simulink model "Pacemaker"  (R2020a)
settings: Solver=FixedStepAuto  StartTime=0.0  StopTime=inf  FixedStep=1e-3  RelTol=1e-3  EnableMultiTasking=on
undefined symbols (not defined in the file): A0, A1, D0, D1, D10, D11, D12, D13, D2, D3, D4, D5, D6, D7, D8, D9, magnitude, PTA0, PTA1, PTA2, PTB2, PTB23, PTB3, PTB9, PTC16, PTC17, PTC2, PTC3, PTC4, PTD0, PTD1, PTD2, PTD3
libraries: frdmk64flib x22, etargetslib x22
settings Model: ExtModeTrigDuration=5  Creator=ffara  LastModifiedBy=Usman Minhas
settings OptimizationCC: EnhancedBackFolding=on  PassReuseOutputArgsAs=Individual arguments  ZeroExternalMemoryAtStartup=off  ZeroInternalMemoryAtStartup=off  MaxStackSize=64  OptimizeBlockOrder=speed  DifferentSizesBufferReuse=on  OptimizationCustomize=off  EfficientTunableParamExpr=on
settings DebuggingCC: ParameterTunabilityLossMsg=error
settings HardwareCC: ProdBitPerPointer=32  ProdBitPerSizeT=32  ProdBitPerPtrDiffT=32  ProdLargestAtomicInteger=Long  ProdLargestAtomicFloat=Double  ProdWordSize=32  ProdHWDeviceType=ARM Compatible->ARM Cortex
settings SFSimCC: MATLABDynamicMemAlloc=off
settings RTWCC: SystemTargetFile=ert.tlc  HardwareBoard=NXP FRDM-K64F  TemplateMakefile=ert_default_tmf  Toolchain=GNU Tools for ARM Embedded Processors
settings CodeAppCC: ForceParamTrailComments=on  IgnoreCustomStorageClasses=off  OperatorAnnotations=on  SimulinkDataObjDesc=on  SFDataObjDesc=on  InsertBlockDesc=on

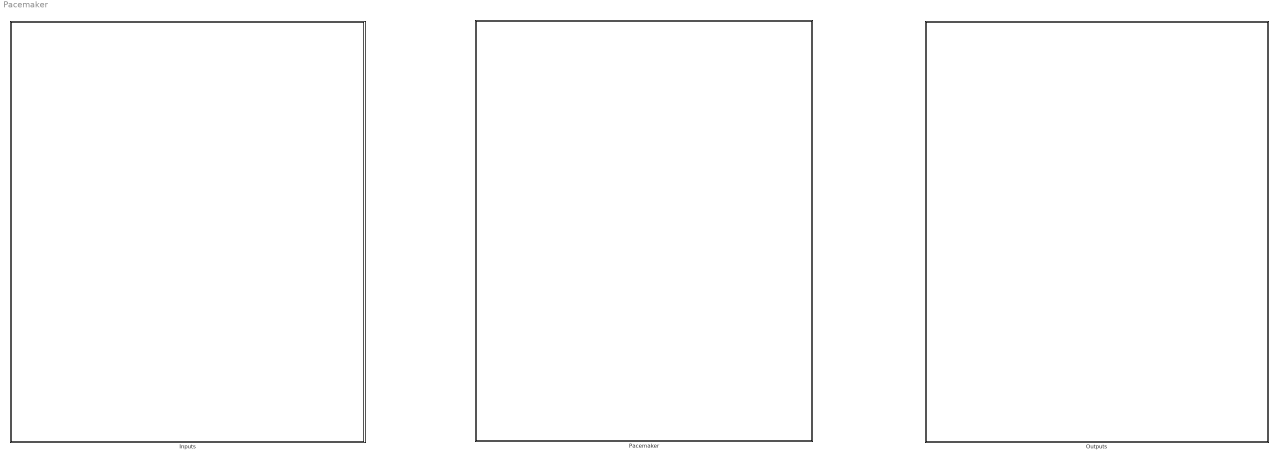
== system Pacemaker ==
  Inputs : Subsystem
  Outputs : Subsystem
  Pacemaker : Subsystem

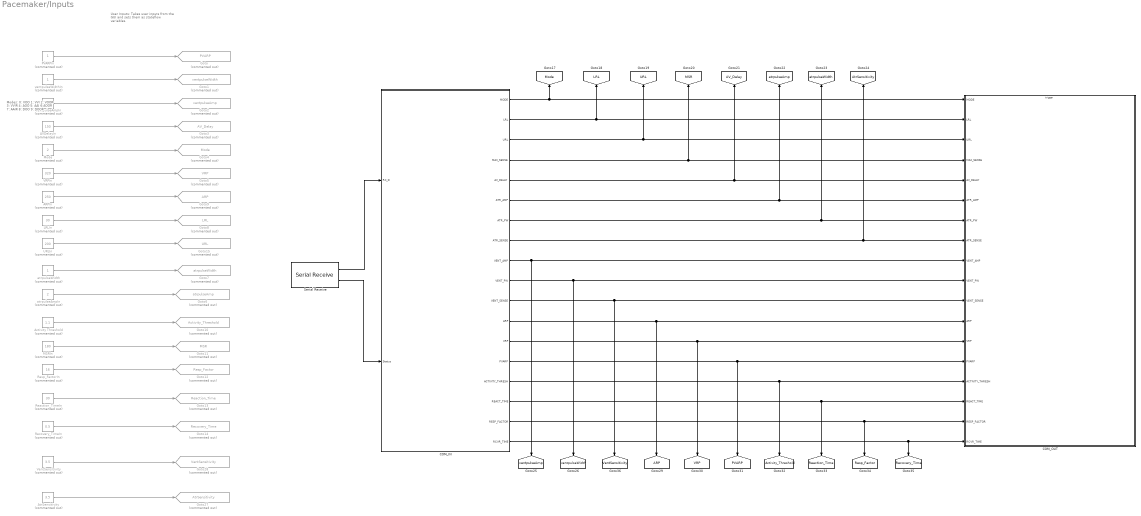
== system Pacemaker/Inputs ==
  note: User Inputs:
      | Takes user inputs from the GUI and sets them as stateflow variables.
  note: Modes:
      | 0: VOO
      | 1: VVI
      | 2: VOOR
      | 3: VVIR
      | 4: AOO
      | 5: AAI
      | 6:AOOR
      | 7: AAIR
      | 8: DOO
      | 9: DOOR
  ARPIn : Constant  Commented=on  Value=250
  AVDelayIn : Constant  Commented=on  Value=150
  Activity Threshold : Constant  Commented=on  Value=1.1
  AtrSensitivity : Constant  Commented=on  Value=3.5
  COM_IN : Stateflow chart  TreatAsAtomicUnit=on
  COM_OUT : Subsystem
  Goto : Goto  Commented=on  GotoTag=PVARP  TagVisibility=global
  Goto1 : Goto  Commented=on  GotoTag=ventpulseWidth  TagVisibility=global
  Goto10 : Goto  Commented=on  GotoTag=Activity_Threshold  TagVisibility=global
  Goto11 : Goto  Commented=on  GotoTag=MSR  TagVisibility=global
  Goto12 : Goto  Commented=on  GotoTag=Resp_Factor  TagVisibility=global
  Goto13 : Goto  Commented=on  GotoTag=Reaction_Time  TagVisibility=global
  Goto14 : Goto  Commented=on  GotoTag=Recovery_Time  TagVisibility=global
  Goto15 : Goto  Commented=on  GotoTag=URL  TagVisibility=global
  Goto2 : Goto  Commented=on  GotoTag=ventpulseAmp  TagVisibility=global
  Goto27 : Goto  Commented=on  GotoTag=AtrSensitivity  TagVisibility=global
  Goto28 : Goto  Commented=on  GotoTag=VentSensitivity  TagVisibility=global
  Goto3 : Goto  Commented=on  GotoTag=AV_Delay  TagVisibility=global
  Goto4 : Goto  Commented=on  GotoTag=Mode  TagVisibility=global
  Goto5 : Goto  Commented=on  GotoTag=VRP  TagVisibility=global
  Goto6 : Goto  Commented=on  GotoTag=atrpulseAmp  TagVisibility=global
  Goto7 : Goto  Commented=on  GotoTag=atrpulseWidth  TagVisibility=global
  Goto8 : Goto  Commented=on  GotoTag=LRL  TagVisibility=global
  Goto9 : Goto  Commented=on  GotoTag=ARP  TagVisibility=global
  LRLIn : Constant  Commented=on  Value=30
  MSRIn : Constant  Commented=on  Value=180
  Mode : Constant  Commented=on  Value=2
  PVARPIn : Constant  Commented=on
  Reaction_TimeIn : Constant  Commented=on  Value=30
  Recovery_TimeIn : Constant  Commented=on  Value=0.5
  Resp_FactorIn : Constant  Commented=on  Value=16
  Serial Receive : frdmk64flib/Serial Receive  SCIModule=0  Baudrate=uint32(9600)  Parity=None  StopBits=1  HardwareFlowControl=None  ByteOrder=LittleEndian  DataType=uint8  DataLength=68  BlockingMode=off  OutputStatus=on  SampleTime=-1
  URLIn : Constant  Commented=on  Value=200
  VRPIn : Constant  Commented=on  Value=320
  VentSensitivity : Constant  Commented=on  Value=3.5
  atrpulseAmpIn : Constant  Commented=on  Value=2
  atrpulseWidth : Constant  Commented=on
  ventpulseAmpIn : Constant  Commented=on  Value=5
  ventpulseWidthIn : Constant  Commented=on
  tag scope: ARP=global, AV_Delay=global, Activity_Threshold=global, AtrSensitivity=global, LRL=global, MSR=global, Mode=global, PVARP=global, Reaction_Time=global, Recovery_Time=global, Resp_Factor=global, URL=global, VRP=global, VentSensitivity=global, atrpulseAmp=global, atrpulseWidth=global, ventpulseAmp=global, ventpulseWidth=global
  wires:
  Resp_FactorIn/1 -> Goto12/1
  PVARPIn/1 -> Goto/1
  VRPIn/1 -> Goto5/1
  ventpulseWidthIn/1 -> Goto1/1
  LRLIn/1 -> Goto8/1
  VentSensitivity/1 -> Goto28/1
  Mode/1 -> Goto4/1
  AtrSensitivity/1 -> Goto27/1
  URLIn/1 -> Goto15/1
  atrpulseWidth/1 -> Goto7/1
  AVDelayIn/1 -> Goto3/1
  ARPIn/1 -> Goto9/1
  atrpulseAmpIn/1 -> Goto6/1
  ventpulseAmpIn/1 -> Goto2/1
  Activity Threshold/1 -> Goto10/1
  Reaction_TimeIn/1 -> Goto13/1
  Recovery_TimeIn/1 -> Goto14/1
  MSRIn/1 -> Goto11/1
  Serial Receive/2 -> COM_IN/2(Status)
  COM_IN/1(MODE) -> [Mode], COM_OUT/1(MODE)
  Serial Receive/1 -> COM_IN/1(RX_D)
  COM_IN/2(LRL) -> [LRL], COM_OUT/2(LRL)
  COM_IN/3(URL) -> [URL], COM_OUT/3(URL)
  COM_IN/4(MAX_SENSE) -> [MSR], COM_OUT/4(MAX_SENSE)
  COM_IN/5(AV_DELAY) -> [AV_Delay], COM_OUT/5(AV_DELAY)
  COM_IN/6(ATR_AMP) -> [atrpulseAmp], COM_OUT/6(ATR_AMP)
  COM_IN/7(ATR_PW) -> [atrpulseWidth], COM_OUT/7(ATR_PW)
  COM_IN/8(ATR_SENSE) -> [AtrSensitivity], COM_OUT/8(ATR_SENSE)
  COM_IN/9(VENT_AMP) -> [ventpulseAmp], COM_OUT/9(VENT_AMP)
  COM_IN/10(VENT_PW) -> COM_OUT/10(VENT_PW), [ventpulseWidth]
  COM_IN/11(VENT_SENSE) -> [VentSensitivity], COM_OUT/11(VENT_SENSE)
  COM_IN/12(ARP) -> COM_OUT/12(ARP), [ARP]
  COM_IN/13(VRP) -> [VRP], COM_OUT/13(VRP)
  COM_IN/14(PVARP) -> [PVARP], COM_OUT/14(PVARP)
  COM_IN/15(ACTIVITY_THRESH) -> [Activity_Threshold], COM_OUT/15(ACTIVITY_THRESH)
  COM_IN/16(REACT_TIME) -> [Reaction_Time], COM_OUT/16(REACT_TIME)
  COM_IN/17(RESP_FACTOR) -> [Resp_Factor], COM_OUT/17(RESP_FACTOR)
  COM_IN/18(RCVR_TIME) -> [Recovery_Time], COM_OUT/18(RCVR_TIME)

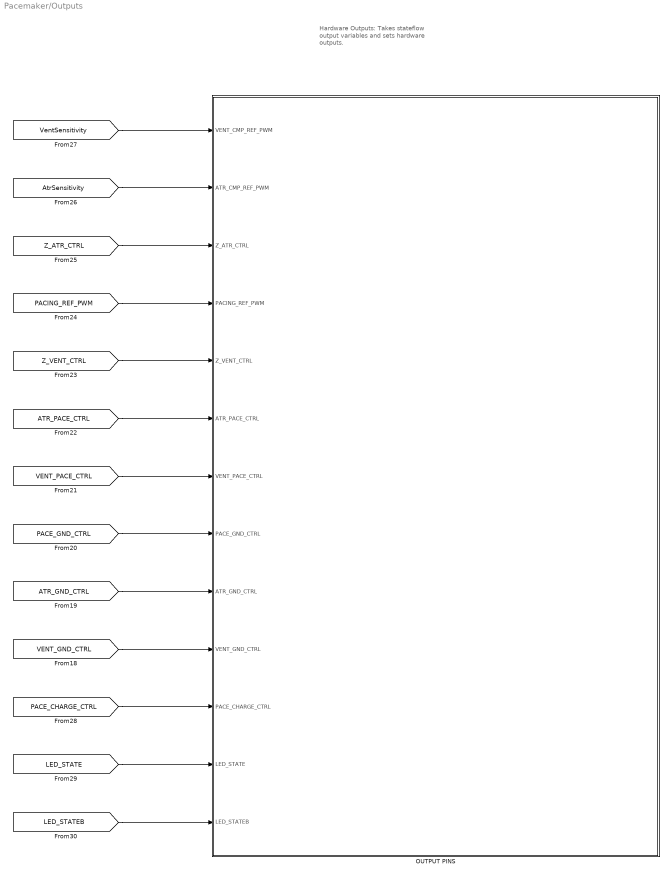
== system Pacemaker/Outputs ==
  note: Hardware Outputs:
      | Takes stateflow output variables and sets hardware outputs.
  OUTPUT PINS : Subsystem
  wires:
  [VentSensitivity] -> OUTPUT PINS/1(VENT_CMP_REF_PWM)
  [PACE_CHARGE_CTRL] -> OUTPUT PINS/11(PACE_CHARGE_CTRL)
  [ATR_PACE_CTRL] -> OUTPUT PINS/6(ATR_PACE_CTRL)
  [LED_STATEB] -> OUTPUT PINS/13(LED_STATEB)
  [LED_STATE] -> OUTPUT PINS/12(LED_STATE)
  [PACING_REF_PWM] -> OUTPUT PINS/4(PACING_REF_PWM)
  [AtrSensitivity] -> OUTPUT PINS/2(ATR_CMP_REF_PWM)
  [Z_ATR_CTRL] -> OUTPUT PINS/3(Z_ATR_CTRL)
  [PACE_GND_CTRL] -> OUTPUT PINS/8(PACE_GND_CTRL)
  [VENT_PACE_CTRL] -> OUTPUT PINS/7(VENT_PACE_CTRL)
  [ATR_GND_CTRL] -> OUTPUT PINS/9(ATR_GND_CTRL)
  [Z_VENT_CTRL] -> OUTPUT PINS/5(Z_VENT_CTRL)
  [VENT_GND_CTRL] -> OUTPUT PINS/10(VENT_GND_CTRL)

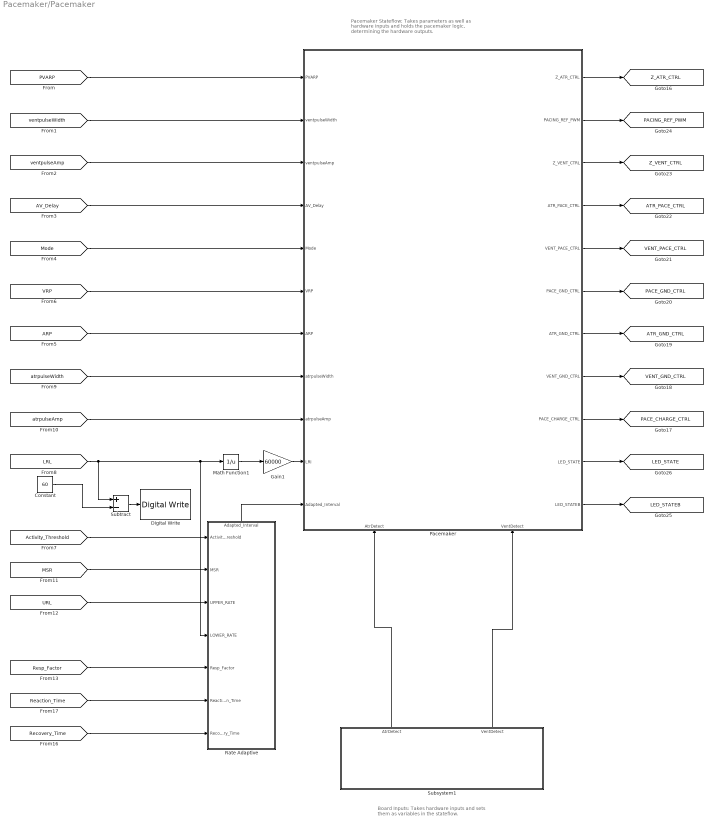
== system Pacemaker/Pacemaker ==
  note: Board Inputs:
      | Takes hardware inputs and sets them as variables in the stateflow.
  note: Pacemaker Stateflow:
      | Takes parameters as well as hardware inputs
      | and holds the pacemaker logic, determining the hardware outputs.
  Constant : Constant  Value=60
  Digital Write : frdmk64flib/Digital Write  Whichpin=GREEN_LED
  Gain1 : Gain  Gain=60000  RndMeth=Ceiling
  Math Function1 : Math  Operator=reciprocal  OutputSignalType=real  OutDataTypeStr=double  RndMeth=Ceiling  SaturateOnIntegerOverflow=on
  Pacemaker : Stateflow chart  TreatAsAtomicUnit=on
      settings: PortSchema="{\"entries\":[{\"content\":{\"sides\":[{\"content\":{\"connectorIds\":[\"In1\",\"In10\",\"In3\",\"In4\",\"In6\",\"In7\",\"In8\",\"In9\",\"In13\",\"In12\",\"In11\"]},\"type\":\"ConnectorPlacement.EquallySpacedRectSide\",\"uuid\":\"aed163b7-0e0a-4c56-a109-22d9582f06bc\"},{\"content\":{\"connectorIds\":[\"Out1\",\"Out3\",\"Out2\",\"Out4\",\"Out5\",\"Out6\",\"Out7\",\"Out8\",\"Out9\",\"Out10\",\"Out11\"],\"side\":\"RIGHT\"},\"type\":\"ConnectorPlacement.EquallySpacedRectSide\",\"uuid\":\"7c994607-95c8-4912-b49a-f01b42451ae0\"},{\"content\":{\"connectorIds\":[],\"side\":\"TOP\"},\"type\":\"ConnectorPlacement.EquallySpacedRectSide\",\"uuid\":\"6d27b0f7-5c71-41f2-b80a-818ae3f7f3ce\"},{\"content\":{\"connectorIds\":[\"In2\",\"In5\"],\"side\":\"BOTTOM\"},\"type\":\"ConnectorPlacement.EquallySpacedRectSide\",\"uuid\":\"17f29399-4528-40af-8d63-94f1f3c418c0\"}]},\"type\":\"ConnectorPlacement.EquallySpacedConnector\",\"uuid\":\"6ca6b560-67cc-4d2d-81f4-cc3fe3468b1a\"}],\"packageUris\":[\"http://schema.mathworks.com/mf0/Connector/19700101\"],\"version\":\"1.0\"}"
  Rate Adaptive : Subsystem
      settings: PortSchema="{\"entries\":[{\"content\":{\"sides\":[{\"content\":{\"connectorIds\":[\"In1\",\"In2\",\"In3\",\"In4\",\"In5\",\"In6\",\"In7\"]},\"type\":\"ConnectorPlacement.EquallySpacedRectSide\",\"uuid\":\"c17ee6c3-7042-4555-a185-2b3f1c7c5c48\"},{\"content\":{\"connectorIds\":[],\"side\":\"RIGHT\"},\"type\":\"ConnectorPlacement.EquallySpacedRectSide\",\"uuid\":\"ce834616-f3de-4ad9-afed-1295335ec238\"},{\"content\":{\"connectorIds\":[\"Out1\"],\"side\":\"TOP\"},\"type\":\"ConnectorPlacement.EquallySpacedRectSide\",\"uuid\":\"ee6be2e3-da9a-4870-9d5e-446ab0e3551d\"}]},\"type\":\"ConnectorPlacement.EquallySpacedConnector\",\"uuid\":\"5402bfdc-705b-4da9-91cb-a8abac72fcc2\"}],\"packageUris\":[\"http://schema.mathworks.com/mf0/Connector/19700101\"],\"version\":\"1.0\"}"
  Subsystem1 : Subsystem
      settings: PortSchema="{\"entries\":[{\"content\":{\"sides\":[{\"content\":{\"connectorIds\":[]},\"type\":\"ConnectorPlacement.EquallySpacedRectSide\",\"uuid\":\"29534348-9b3e-49a9-890e-1782155d7d1f\"},{\"content\":{\"connectorIds\":[],\"side\":\"RIGHT\"},\"type\":\"ConnectorPlacement.EquallySpacedRectSide\",\"uuid\":\"db3d28f5-8266-45b6-9ee4-e43788b67d28\"},{\"content\":{\"connectorIds\":[\"Out1\",\"Out2\"],\"side\":\"TOP\"},\"type\":\"ConnectorPlacement.EquallySpacedRectSide\",\"uuid\":\"67bf6cf6-8ed6-4181-b5d9-914949d467ab\"}]},\"type\":\"ConnectorPlacement.EquallySpacedConnector\",\"uuid\":\"34dda7e8-1d86-47a2-be1a-f2253f8f1257\"}],\"packageUris\":[\"http://schema.mathworks.com/mf0/Connector/R2020b\"],\"version\":\"1.0\"}"
  Subtract : Sum  Inputs=+-
  tag scope: ATR_GND_CTRL=global, ATR_PACE_CTRL=global, LED_STATE=global, LED_STATEB=global, PACE_CHARGE_CTRL=global, PACE_GND_CTRL=global, PACING_REF_PWM=global, VENT_GND_CTRL=global, VENT_PACE_CTRL=global, Z_ATR_CTRL=global, Z_VENT_CTRL=global
  wires:
  Pacemaker/7(ATR_GND_CTRL) -> [ATR_GND_CTRL]
  Subsystem1/1(AtrDetect) -> Pacemaker/2(AtrDetect)
  Pacemaker/4(ATR_PACE_CTRL) -> [ATR_PACE_CTRL]
  Pacemaker/10(LED_STATE) -> [LED_STATE]
  [AV_Delay] -> Pacemaker/4(AV_Delay)
  Pacemaker/2(Z_VENT_CTRL) -> [Z_VENT_CTRL]
  [Mode] -> Pacemaker/6(Mode)
  [ARP] -> Pacemaker/8(ARP)
  Pacemaker/1(Z_ATR_CTRL) -> [Z_ATR_CTRL]
  Math Function1/1 -> Gain1/1
  [atrpulseWidth] -> Pacemaker/9(atrpulseWidth)
  [PVARP] -> Pacemaker/1(PVARP)
  Pacemaker/5(VENT_PACE_CTRL) -> [VENT_PACE_CTRL]
  Pacemaker/6(PACE_GND_CTRL) -> [PACE_GND_CTRL]
  Pacemaker/11(LED_STATEB) -> [LED_STATEB]
  [Resp_Factor] -> Rate Adaptive/5(Resp_Factor)
  Pacemaker/3(PACING_REF_PWM) -> [PACING_REF_PWM]
  [MSR] -> Rate Adaptive/2(MSR)
  [ventpulseWidth] -> Pacemaker/10(ventpulseWidth)
  Pacemaker/8(VENT_GND_CTRL) -> [VENT_GND_CTRL]
  Pacemaker/9(PACE_CHARGE_CTRL) -> [PACE_CHARGE_CTRL]
  [ventpulseAmp] -> Pacemaker/3(ventpulseAmp)
  [Recovery_Time] -> Rate Adaptive/7(Recovery_Time)
  Subsystem1/2(VentDetect) -> Pacemaker/5(VentDetect)
  [URL] -> Rate Adaptive/3(UPPER_RATE)
  [atrpulseAmp] -> Pacemaker/13(atrpulseAmp)
  Gain1/1 -> Pacemaker/12(LRI)
  [VRP] -> Pacemaker/7(VRP)
  [Activity_Threshold] -> Rate Adaptive/1(Activity_Threshold)
  [LRL] -> Subtract/1, Math Function1/1, Rate Adaptive/4(LOWER_RATE)
  Rate Adaptive/1(Adapted_Interval) -> Pacemaker/11(Adapted_Interval)
  [Reaction_Time] -> Rate Adaptive/6(Reaction_Time)
  Subtract/1 -> Digital Write/1
  Constant/1 -> Subtract/2

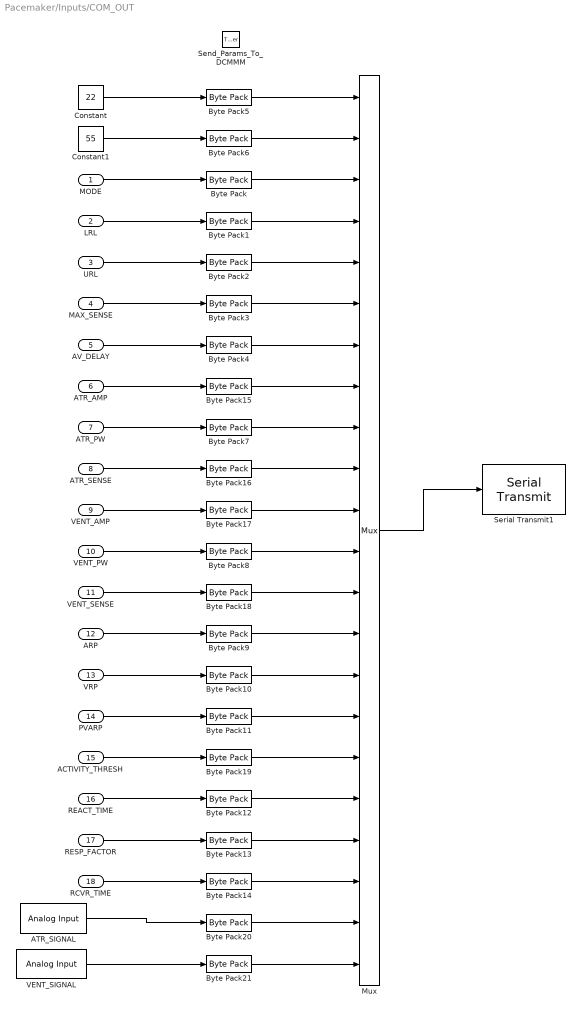
== system Pacemaker/Inputs/COM_OUT ==
  MODE : Inport
  LRL : Inport  Port=2
  URL : Inport  Port=3
  MAX_SENSE : Inport  Port=4
  AV_DELAY : Inport  Port=5
  ATR_AMP : Inport  Port=6
  ATR_PW : Inport  Port=7
  ATR_SENSE : Inport  Port=8
  VENT_AMP : Inport  Port=9
  VENT_PW : Inport  Port=10
  VENT_SENSE : Inport  Port=11
  ARP : Inport  Port=12
  VRP : Inport  Port=13
  PVARP : Inport  Port=14
  ACTIVITY_THRESH : Inport  Port=15
  REACT_TIME : Inport  Port=16
  RESP_FACTOR : Inport  Port=17
  RCVR_TIME : Inport  Port=18
  Send_Params_To_DCMMM : TriggerPort  TriggerType=function-call  IsSimulinkFunction=on  FunctionName=Send_Params_To_DCMMM  VariantControl=Variant
  ATR_SIGNAL : frdmk64flib/Analog Input  Whichpin=PTB2 (A0)  SampleTime=-1
  Byte Pack{,1..4,7..14} (13 alike) : etargetslib/Byte Pack  datatypes={'uint16'}  byteAlign=1
  Byte Pack{15..21} (7 alike) : etargetslib/Byte Pack  datatypes={'double'}  byteAlign=1
  Byte Pack5 : etargetslib/Byte Pack  datatypes={'uint8'}  byteAlign=1
  Byte Pack6 : etargetslib/Byte Pack  datatypes={'uint8'}  byteAlign=1
  Constant : Constant  Value=22  OutDataTypeStr=uint8
  Constant1 : Constant  Value=55  OutDataTypeStr=uint8
  Mux : Mux  Inputs=22
  Serial Transmit1 : frdmk64flib/Serial Transmit  SCIModule=0  Baudrate=uint32(9600)  Parity=None  StopBits=1  HardwareFlowControl=None  ByteOrder=LittleEndian  BlockingMode=on  OutputStatus=off
  VENT_SIGNAL : frdmk64flib/Analog Input  Whichpin=PTB3 (A1)  SampleTime=-1
  wires:
  Mux/1 -> Serial Transmit1/1
  MODE/1 -> Byte Pack/1
  Byte Pack/1 -> Mux/3
  Constant/1 -> Byte Pack5/1
  Byte Pack5/1 -> Mux/1
  Byte Pack6/1 -> Mux/2
  Constant1/1 -> Byte Pack6/1
  Byte Pack1/1 -> Mux/4
  Byte Pack2/1 -> Mux/5
  Byte Pack3/1 -> Mux/6
  Byte Pack4/1 -> Mux/7
  URL/1 -> Byte Pack2/1
  MAX_SENSE/1 -> Byte Pack3/1
  AV_DELAY/1 -> Byte Pack4/1
  RCVR_TIME/1 -> Byte Pack14/1
  RESP_FACTOR/1 -> Byte Pack13/1
  REACT_TIME/1 -> Byte Pack12/1
  Byte Pack12/1 -> Mux/18
  Byte Pack13/1 -> Mux/19
  Byte Pack14/1 -> Mux/20
  Byte Pack9/1 -> Mux/14
  Byte Pack10/1 -> Mux/15
  Byte Pack11/1 -> Mux/16
  PVARP/1 -> Byte Pack11/1
  VRP/1 -> Byte Pack10/1
  ARP/1 -> Byte Pack9/1
  Byte Pack7/1 -> Mux/9
  Byte Pack8/1 -> Mux/12
  VENT_PW/1 -> Byte Pack8/1
  ATR_PW/1 -> Byte Pack7/1
  LRL/1 -> Byte Pack1/1
  Byte Pack19/1 -> Mux/17
  Byte Pack17/1 -> Mux/11
  Byte Pack16/1 -> Mux/10
  Byte Pack15/1 -> Mux/8
  Byte Pack18/1 -> Mux/13
  ATR_AMP/1 -> Byte Pack15/1
  ATR_SENSE/1 -> Byte Pack16/1
  VENT_AMP/1 -> Byte Pack17/1
  VENT_SENSE/1 -> Byte Pack18/1
  ACTIVITY_THRESH/1 -> Byte Pack19/1
  ATR_SIGNAL/1 -> Byte Pack20/1
  VENT_SIGNAL/1 -> Byte Pack21/1
  Byte Pack20/1 -> Mux/21
  Byte Pack21/1 -> Mux/22

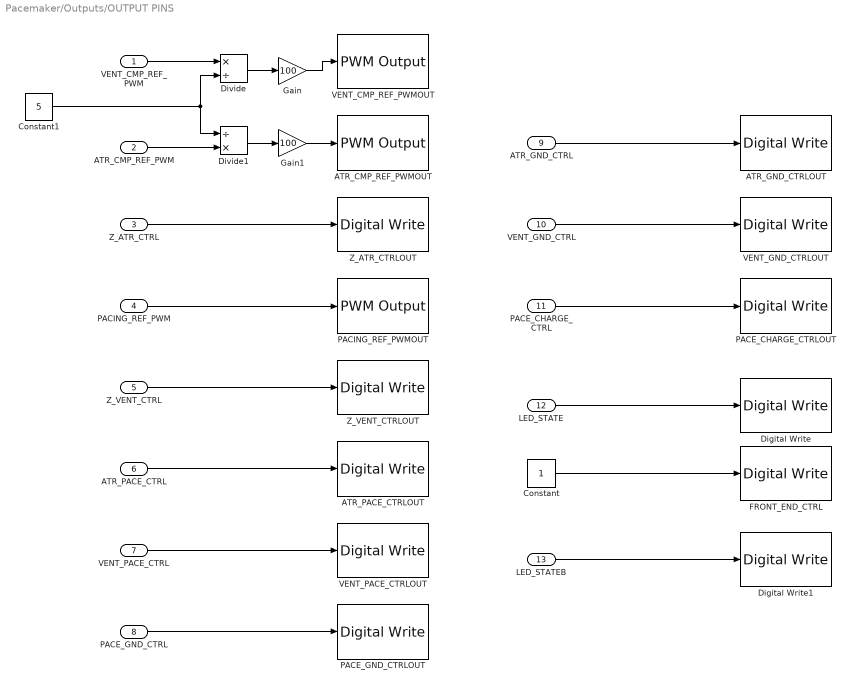
== system Pacemaker/Outputs/OUTPUT PINS ==
  VENT_CMP_REF_PWM : Inport  Unit=mV
  ATR_CMP_REF_PWM : Inport  Port=2  Unit=mV
  Z_ATR_CTRL : Inport  Port=3
  PACING_REF_PWM : Inport  Port=4
  Z_VENT_CTRL : Inport  Port=5
  ATR_PACE_CTRL : Inport  Port=6
  VENT_PACE_CTRL : Inport  Port=7
  PACE_GND_CTRL : Inport  Port=8
  ATR_GND_CTRL : Inport  Port=9
  VENT_GND_CTRL : Inport  Port=10
  PACE_CHARGE_CTRL : Inport  Port=11
  LED_STATE : Inport  Port=12
  LED_STATEB : Inport  Port=13
  ATR_CMP_REF_PWMOUT : frdmk64flib/PWM Output  Whichpin=PTC2 (D6)  InitialFrequency=2000  InitialDutyCycle=0
  ATR_GND_CTRLOUT : frdmk64flib/Digital Write  Whichpin=PTD2 (D11)
  ATR_PACE_CTRLOUT : frdmk64flib/Digital Write  Whichpin=PTA0 (D8)
  Constant : Constant
  Constant1 : Constant  Value=5
  Digital Write : frdmk64flib/Digital Write  Whichpin=RED_LED
  Digital Write1 : frdmk64flib/Digital Write  Whichpin=BLUE_LED
  Divide : Product  Inputs=*/
  Divide1 : Product  Inputs=/*
  FRONT_END_CTRL : frdmk64flib/Digital Write  Whichpin=PTD1 (D13)
  Gain : Gain  Gain=100
  Gain1 : Gain  Gain=100
  PACE_CHARGE_CTRLOUT : frdmk64flib/Digital Write  Whichpin=PTB9 (D2)
  PACE_GND_CTRLOUT : frdmk64flib/Digital Write  Whichpin=PTD0 (D10)
  PACING_REF_PWMOUT : frdmk64flib/PWM Output  Whichpin=PTA2 (D5)  InitialFrequency=2000  InitialDutyCycle=0
  VENT_CMP_REF_PWMOUT : frdmk64flib/PWM Output  Whichpin=PTA1 (D3)  InitialFrequency=2000  InitialDutyCycle=0
  VENT_GND_CTRLOUT : frdmk64flib/Digital Write  Whichpin=PTD3 (D12)
  VENT_PACE_CTRLOUT : frdmk64flib/Digital Write  Whichpin=PTC4 (D9)
  Z_ATR_CTRLOUT : frdmk64flib/Digital Write  Whichpin=PTB23 (D4)
  Z_VENT_CTRLOUT : frdmk64flib/Digital Write  Whichpin=PTC3 (D7)
  wires:
  PACE_CHARGE_CTRL/1 -> PACE_CHARGE_CTRLOUT/1
  PACE_GND_CTRL/1 -> PACE_GND_CTRLOUT/1
  ATR_GND_CTRL/1 -> ATR_GND_CTRLOUT/1
  VENT_PACE_CTRL/1 -> VENT_PACE_CTRLOUT/1
  ATR_PACE_CTRL/1 -> ATR_PACE_CTRLOUT/1
  Z_VENT_CTRL/1 -> Z_VENT_CTRLOUT/1
  VENT_GND_CTRL/1 -> VENT_GND_CTRLOUT/1
  PACING_REF_PWM/1 -> PACING_REF_PWMOUT/1
  Z_ATR_CTRL/1 -> Z_ATR_CTRLOUT/1
  LED_STATE/1 -> Digital Write/1
  ATR_CMP_REF_PWM/1 -> Divide1/2
  Constant/1 -> FRONT_END_CTRL/1
  LED_STATEB/1 -> Digital Write1/1
  VENT_CMP_REF_PWM/1 -> Divide/1
  Constant1/1 -> Divide1/1, Divide/2
  Divide/1 -> Gain/1
  Gain/1 -> VENT_CMP_REF_PWMOUT/1
  Divide1/1 -> Gain1/1
  Gain1/1 -> ATR_CMP_REF_PWMOUT/1

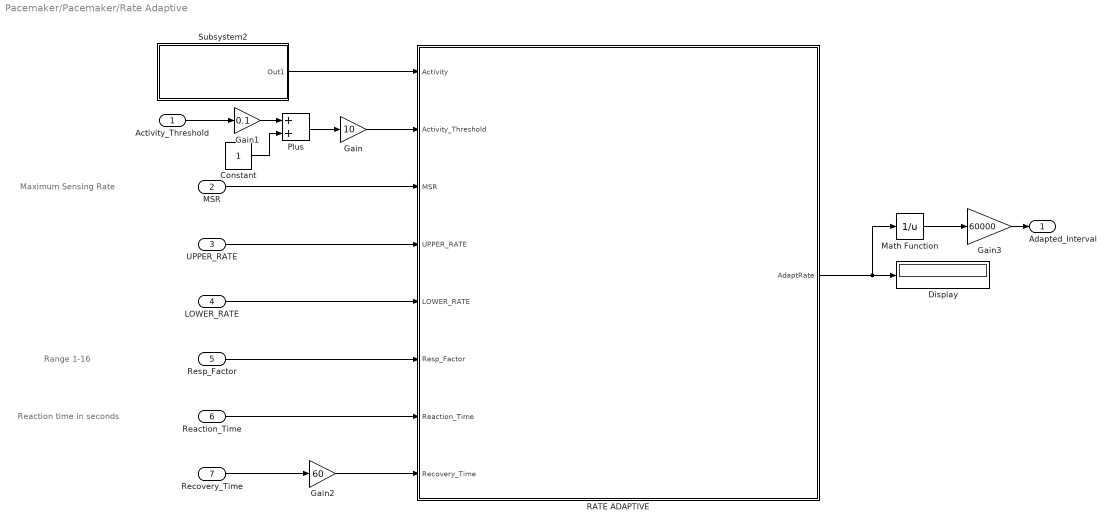
== system Pacemaker/Pacemaker/Rate Adaptive ==
  note: Range 1-16
  note: Reaction time in seconds
  note: Maximum Sensing Rate
  Activity_Threshold : Inport
  MSR : Inport  Port=2
  UPPER_RATE : Inport  Port=3
  LOWER_RATE : Inport  Port=4
  Resp_Factor : Inport  Port=5
  Reaction_Time : Inport  Port=6
  Recovery_Time : Inport  Port=7
  Constant : Constant
  Display : Display
  Gain : Gain  Gain=10  OutDataTypeStr=double  RndMeth=Ceiling
  Gain1 : Gain  Gain=0.1
  Gain2 : Gain  Gain=60
  Gain3 : Gain  Gain=60000
  Math Function : Math  Operator=reciprocal  OutputSignalType=real  OutDataTypeStr=double  RndMeth=Ceiling  SaturateOnIntegerOverflow=on
  Plus : Sum
  RATE ADAPTIVE : Stateflow chart  TreatAsAtomicUnit=on
  Subsystem2 : Subsystem
  Adapted_Interval : Outport
  wires:
  RATE ADAPTIVE/1(AdaptRate) -> Math Function/1, Display/1
  Recovery_Time/1 -> Gain2/1
  Gain2/1 -> RATE ADAPTIVE/8(Recovery_Time)
  Resp_Factor/1 -> RATE ADAPTIVE/6(Resp_Factor)
  Math Function/1 -> Gain3/1
  Gain/1 -> RATE ADAPTIVE/2(Activity_Threshold)
  Subsystem2/1(Out1) -> RATE ADAPTIVE/1(Activity)
  Gain3/1 -> Adapted_Interval/1
  Activity_Threshold/1 -> Gain1/1
  MSR/1 -> RATE ADAPTIVE/3(MSR)
  UPPER_RATE/1 -> RATE ADAPTIVE/4(UPPER_RATE)
  LOWER_RATE/1 -> RATE ADAPTIVE/5(LOWER_RATE)
  Reaction_Time/1 -> RATE ADAPTIVE/7(Reaction_Time)
  Gain1/1 -> Plus/1
  Plus/1 -> Gain/1
  Constant/1 -> Plus/2

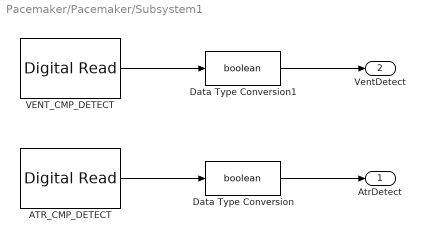
== system Pacemaker/Pacemaker/Subsystem1 ==
  ATR_CMP_DETECT : frdmk64flib/Digital Read  Whichpin=PTC16 (D0)  SampleTime=-1
  Data Type Conversion : DataTypeConversion  OutDataTypeStr=boolean  RndMeth=Round
  Data Type Conversion1 : DataTypeConversion  OutDataTypeStr=boolean  RndMeth=Round
  VENT_CMP_DETECT : frdmk64flib/Digital Read  Whichpin=PTC17 (D1)  SampleTime=-1
  AtrDetect : Outport
  VentDetect : Outport  Port=2
  wires:
  ATR_CMP_DETECT/1 -> Data Type Conversion/1
  Data Type Conversion/1 -> AtrDetect/1
  Data Type Conversion1/1 -> VentDetect/1
  VENT_CMP_DETECT/1 -> Data Type Conversion1/1

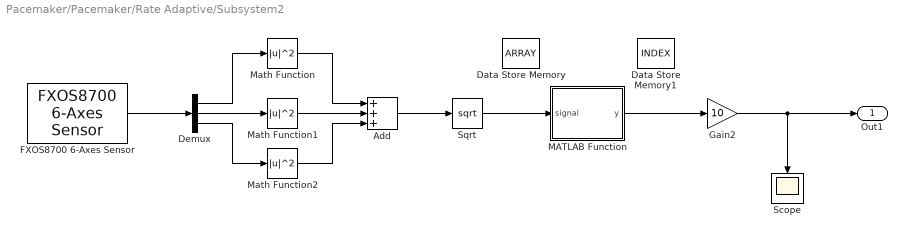
== system Pacemaker/Pacemaker/Rate Adaptive/Subsystem2 ==
  Add : Sum  Inputs=+++
  Data Store Memory : DataStoreMemory  DataStoreName=ARRAY  ReadBeforeWriteMsg=warning  WriteAfterWriteMsg=warning  WriteAfterReadMsg=warning  InitialValue=[1,1,1,1,1,1,1,1,1,1,1,1,1,1,1,1,1,1,1,1,1,1,1,1,1,1,1,1,1,1,1,1,1,1,1,1,1,1,1,1,1,1,1,1,1,1,1,1,1,1]  ShowAdditionalParam=off  OutDataTypeStr=double
  Data Store Memory1 : DataStoreMemory  DataStoreName=INDEX  ReadBeforeWriteMsg=warning  WriteAfterWriteMsg=warning  WriteAfterReadMsg=warning  ShowAdditionalParam=off  OutDataTypeStr=uint8
  Demux : Demux  Outputs=3
  FXOS8700 6-Axes Sensor : frdmk64flib/FXOS8700 6-Axes Sensor  Activesensor=Accelerometer only  ODR=100Hz  HybridODR=400Hz  Accelfullrange=-8g to +8g  SampleTime=0.01
  Gain2 : Gain  Gain=10  OutDataTypeStr=double  RndMeth=Ceiling
  MATLAB Function : MATLAB Function  TreatAsAtomicUnit=on
  Math Function : Math  Operator=magnitude^2  SaturateOnIntegerOverflow=on
  Math Function1 : Math  Operator=magnitude^2  SaturateOnIntegerOverflow=on
  Math Function2 : Math  Operator=magnitude^2  SaturateOnIntegerOverflow=on
  Scope : Scope
  Sqrt : Sqrt  SaturateOnIntegerOverflow=on
  Out1 : Outport
  wires:
  Math Function1/1 -> Add/2
  Add/1 -> Sqrt/1
  Math Function/1 -> Add/1
  Math Function2/1 -> Add/3
  Demux/3 -> Math Function2/1
  MATLAB Function/1(y) -> Gain2/1
  Gain2/1 -> Out1/1, Scope/1
  Demux/2 -> Math Function1/1
  Demux/1 -> Math Function/1
  FXOS8700 6-Axes Sensor/1 -> Demux/1
  Sqrt/1 -> MATLAB Function/1(signal)

== stateflow chart Pacemaker/Rate Adaptive/RATE ADAPTIVE ==
  note: C is a constant that changes according to the Activity_Threshold.
      | It increases so that MSR can always be reached at the max activity level which was found by shaking as hard as possible.
      | Meaning that we do not have to vigorously shake the board to get our target to increase
      | It will scale with response factor and the constant.
  state Stepping_Up
    entry:
    AdaptRate=AdaptRate+StepUp;
    Target=LOWER_RATE+C*Resp_Factor*(double(Activity-Activity_Threshold))
    StepUp=ceil((double(MSR)-double(LOWER_RATE))/double(Reaction_Time))
    StepDown=ceil(double(MSR)-double(LOWER_RATE))/double(Recovery_Time)
  state Halt_Adapt
    entry:AdaptRate=double(UPPER_RATE);
    StepUp=ceil((double(MSR)-double(LOWER_RATE))/double(Reaction_Time))
    StepDown=ceil(double(MSR)-double(LOWER_RATE))/double(Recovery_Time)
    during:Target=LOWER_RATE+C*Resp_Factor*(double(Activity-Activity_Threshold))
  state Start
    Target=LOWER_RATE+C*Resp_Factor*(double(Activity-Activity_Threshold))
    entry:
    StepUp=ceil((double(MSR)-double(LOWER_RATE))/double(Reaction_Time))
    StepDown=ceil(double(MSR)-double(LOWER_RATE))/double(Recovery_Time)
    AdaptRate=double(LOWER_RATE)
    CurrentLRL=double(LOWER_RATE)
  state Finished_Adapt
    entry: AdaptRate=double(MSR);
    StepUp=ceil((double(MSR)-double(LOWER_RATE))/double(Reaction_Time))
    StepDown=ceil(double(MSR)-double(LOWER_RATE))/double(Recovery_Time)
    during:Target=LOWER_RATE+C*Resp_Factor*(double(Activity-Activity_Threshold))
  state Stepping_Down
    entry:
    StepUp=ceil((double(MSR)-double(LOWER_RATE))/double(Reaction_Time))
    StepDown=ceil(double(MSR)-double(LOWER_RATE))/double(Recovery_Time)
    AdaptRate=AdaptRate-StepDown;
    Target=LOWER_RATE+C*Resp_Factor*(double(Activity-Activity_Threshold))
  Halt_Adapt -> Start [order 2] : [CurrentLRL~=LOWER_RATE]
  Stepping_Up -> Stepping_Up [order 1] : after(1,sec)[AdaptRate<Target]
  (default) -> Start : {C=(double(MSR)-double(LOWER_RATE))/(20.0-double(Activity_Threshold))}
  Stepping_Up -> Halt_Adapt [order 3] : [AdaptRate>=UPPER_RATE]
  Stepping_Up -> Start [order 5] : [CurrentLRL~=LOWER_RATE]
  Halt_Adapt -> (junction 35) [order 1] : [Target<UPPER_RATE]
  Start -> Stepping_Up [order 1] : [AdaptRate<Target]
  Stepping_Up -> Stepping_Down [order 4] : after(1,sec)[AdaptRate>Target]
  Stepping_Down -> Stepping_Up [order 3] : after(1,sec)[AdaptRate<Target]
  Stepping_Up -> Finished_Adapt [order 2] : [AdaptRate>=MSR]
  Start -> Start [order 2] : [CurrentLRL~=LOWER_RATE]
  Stepping_Down -> Start [order 2] : [AdaptRate<=LOWER_RATE]
  Stepping_Down -> Start [order 4] : [CurrentLRL~=LOWER_RATE]
  Finished_Adapt -> Start [order 2] : [CurrentLRL~=LOWER_RATE]
  Finished_Adapt -> (junction 35) [order 1] : [Target<MSR]
  (junction 35) -> Stepping_Down
  Stepping_Down -> Stepping_Down [order 1] : after(1,sec)[AdaptRate>Target]
  data: Activity input; Activity_Threshold input; MSR input; UPPER_RATE input; LOWER_RATE input; Resp_Factor input; Reaction_Time input; Recovery_Time input; AdaptRate output; StepUp local; StepDown local; Target local; C local; CurrentLRL local

== matlab function Pacemaker/Rate Adaptive/Subsystem2/MATLAB Function ==
  data: signal input double; y output double; ARRAY data_store_memory; INDEX data_store_memory
function y = fcn(signal)
global INDEX;
INDEX = mod(INDEX + 1, 50) + 1;
global ARRAY;
ARRAY(INDEX) = signal;
y = mean(ARRAY);

== stateflow chart Pacemaker/Pacemaker ==
  note: DOO:
      | Paces the atrium and the ventricle without sensing.
      | First atrium is paced followed by the ventricle after the
      | AV Delay to meet LRL
  note: DOOR:
      | Paces the atrium and the ventricle without sensing.
      | First atrium is paced followed by the ventricle after the
      | AV Delay to meet adapted rate
  state DOO
    state ATR_DISCHARGING
      entry:
      %Discharge C22 into ATR
      %Charge C21
      PACE_CHARGE_CTRL = false
      PACE_GND_CTRL = true
      ATR_PACE_CTRL = true
      ATR_GND_CTRL = false
      Z_ATR_CTRL = false
      Z_VENT_CTRL = false
      VENT_GND_CTRL = false
      VENT_PACE_CTRL = false
    state VENT_CHARGING
      entry:
      %Charge C22
      ATR_PACE_CTRL = false
      VENT_PACE_CTRL = false
      PACING_REF_PWM = ventpulseAmp/5*100;
      PACE_CHARGE_CTRL = true
      %Discharge C21
      PACE_GND_CTRL = true
      VENT_PACE_CTRL = false
      Z_ATR_CTRL = false
      Z_VENT_CTRL = false
      ATR_PACE_CTRL = false
      ATR_GND_CTRL = true
      VENT_GND_CTRL = false
    note: Paces atrium for duration of atrial pulse width
        | after LRI - AV Delay - Ventrical Pulse Width or LRI from
        | rising edge of the last atrium pace
    note: Removes excessvoltage from atrium and begins charging ventricle
    state ATR_CHARGING
      entry:
      %Charge C22
      ATR_PACE_CTRL = false
      VENT_PACE_CTRL = false
      PACING_REF_PWM = atrpulseAmp/5*100;
      PACE_CHARGE_CTRL = true
      %Discharge C21
      PACE_GND_CTRL = true
      VENT_PACE_CTRL = false
      Z_ATR_CTRL = false
      Z_VENT_CTRL = false
      ATR_PACE_CTRL = false
      ATR_GND_CTRL = false
      VENT_GND_CTRL = true
    state VENT_DISCHARGING
      entry:
      %Discharge C22 into VENT
      %Charge C21
      PACE_CHARGE_CTRL = false
      PACE_GND_CTRL = true
      ATR_PACE_CTRL = false
      ATR_GND_CTRL = false
      Z_ATR_CTRL = false
      Z_VENT_CTRL = false
      VENT_GND_CTRL = false
      VENT_PACE_CTRL = true
    note: Delivers ventricle pace for duration of centricle pulse width
        | after AV_Delay has been met
    note: Charges atrium capacitor while draining previous ventrical pace
    note: Checks if mode has changed
    DOO.ATR_DISCHARGING -> DOO.VENT_CHARGING : after(atrpulseWidth,msec)
    DOO.VENT_CHARGING -> DOO.VENT_DISCHARGING : after(AV_Delay - atrpulseWidth, msec)
    (junction 447) -> DOO.ATR_DISCHARGING : after(LRI - AV_Delay - ventpulseWidth, msec)
    DOO.ATR_CHARGING -> (junction 447) [order 2] : [Mode == 8]
    DOO.VENT_DISCHARGING -> DOO.ATR_CHARGING : after(ventpulseWidth,msec)
    (default) -> DOO.ATR_CHARGING
  state DOOR
    state ATR_DISCHARGING
      entry:
      %Discharge C22 into ATR
      %Charge C21
      PACE_CHARGE_CTRL = false
      PACE_GND_CTRL = true
      ATR_PACE_CTRL = true
      ATR_GND_CTRL = false
      Z_ATR_CTRL = false
      Z_VENT_CTRL = false
      VENT_GND_CTRL = false
      VENT_PACE_CTRL = false
    state VENT_CHARGING
      entry:
      %Charge C22
      ATR_PACE_CTRL = false
      VENT_PACE_CTRL = false
      PACING_REF_PWM = ventpulseAmp/5*100;
      PACE_CHARGE_CTRL = true
      %Discharge C21
      PACE_GND_CTRL = true
      VENT_PACE_CTRL = false
      Z_ATR_CTRL = false
      Z_VENT_CTRL = false
      ATR_PACE_CTRL = false
      ATR_GND_CTRL = true
      VENT_GND_CTRL = false
    note: Paces atrium for duration of atrial pulse width
        | after Adapted_Interval - AV Delay - Ventrical Pulse Width or LRI from
        | rising edge of the last atrium pace
    note: Removes excessvoltage from atrium and begins charging ventricle
    state ATR_CHARGING
      entry:
      %Charge C22
      ATR_PACE_CTRL = false
      VENT_PACE_CTRL = false
      PACING_REF_PWM = atrpulseAmp/5*100;
      PACE_CHARGE_CTRL = true
      %Discharge C21
      PACE_GND_CTRL = true
      VENT_PACE_CTRL = false
      Z_ATR_CTRL = false
      Z_VENT_CTRL = false
      ATR_PACE_CTRL = false
      ATR_GND_CTRL = false
      VENT_GND_CTRL = true
    state VENT_DISCHARGING
      entry:
      %Discharge C22 into VENT
      %Charge C21
      PACE_CHARGE_CTRL = false
      PACE_GND_CTRL = true
      ATR_PACE_CTRL = false
      ATR_GND_CTRL = false
      Z_ATR_CTRL = false
      Z_VENT_CTRL = false
      VENT_GND_CTRL = false
      VENT_PACE_CTRL = true
    note: Delivers ventricle pace for duration of centricle pulse width
        | after AV_Delay has been met
    note: Charges atrium capacitor while draining previous ventrical pace
    note: Checks if mode has changed
    DOOR.ATR_DISCHARGING -> DOOR.VENT_CHARGING : after(atrpulseWidth,msec)
    DOOR.VENT_CHARGING -> DOOR.VENT_DISCHARGING : after(AV_Delay - atrpulseWidth, msec)
    (junction 449) -> DOOR.ATR_DISCHARGING : after(Adapted_Interval - AV_Delay - ventpulseWidth, msec)
    DOOR.ATR_CHARGING -> (junction 449) [order 2] : [Mode == 9]
    DOOR.VENT_DISCHARGING -> DOOR.ATR_CHARGING : after(ventpulseWidth,msec)
    (default) -> DOOR.ATR_CHARGING
  state INITIALIZER
    entry:
    if Mode<=3
    PACING_REF_PWM=ventpulseAmp/5*100;
    else
    PACING_REF_PWM=atrpulseAmp/5*100;
    end
    note: Initializer:
        | Sets up the pins required as well as the PWM frequency then moves to a state based on the mode specified.
  state AOOR
    note: Checks if mode has changed
    state Charging
      entry:
      %discharge C21 first
      PACE_GND_CTRL=true;
      VENT_PACE_CTRL=false;
      Z_ATR_CTRL=false;
      Z_VENT_CTRL=false;
      ATR_PACE_CTRL=false;
      ATR_GND_CTRL=true;
      VENT_GND_CTRL=false;
      %charging C22
      PACING_REF_PWM=atrpulseAmp/5*100;%input from GUI
      PACE_CHARGE_CTRL=true;
    state Pacing
      entry:
      PACE_CHARGE_CTRL=false;
      PACE_GND_CTRL=true;
      ATR_PACE_CTRL=true;
      ATR_GND_CTRL=false;
      Z_ATR_CTRL=false;
      Z_VENT_CTRL=false;
      VENT_GND_CTRL=false;
      VENT_PACE_CTRL=false;
    note: Drains excess current from heart and delivers next pace after the adapted interval
        | in order to meet the adapted rate limit
    note: Paces atrium for duration of pulse width
    (default) -> AOOR.Charging
    AOOR.Pacing -> AOOR.Charging : after(atrpulseWidth,msec)
    AOOR.Charging -> (junction 445) [order 2] : [Mode==6]
    (junction 445) -> AOOR.Pacing : after(Adapted_Interval-atrpulseWidth,msec)
  note: AOOR:
      | Atrial pacing at adapted rate through discharging C22, discharging C21, and recharging C22.
  note: VOOR:
      | Ventricular pacing at adapted rate through discharging C22, discharging C21, and recharging C22.
  state VOOR
    note: Checks if mode has changed
    state Charging
      entry:
      %discharge C21 first at VENT_GND
      PACE_GND_CTRL=true;
      VENT_PACE_CTRL=false;
      Z_ATR_CTRL=false;
      Z_VENT_CTRL=false;
      ATR_PACE_CTRL=false;
      ATR_GND_CTRL=false;
      VENT_GND_CTRL=true;
      %charging C22
      %input from GUI
      PACING_REF_PWM=ventpulseAmp/5*100;
      PACE_CHARGE_CTRL=true;
      LED_STATE=true;
    state Pacing
      entry:
      %discharging C22 at VENT
      PACE_CHARGE_CTRL=false;
      PACE_GND_CTRL=true;
      ATR_PACE_CTRL=false;
      ATR_GND_CTRL=false;
      Z_ATR_CTRL=false;
      Z_VENT_CTRL=false;
      VENT_GND_CTRL=false;
      VENT_PACE_CTRL=true;
      LED_STATE=false;
    note: Drains excess current from heart and delivers
        |  pace after Adapted Interval to meet Adapted Rate Limit
    note: Delivers pulse to ventricle for duration of pulse width
    (default) -> VOOR.Charging
    VOOR.Pacing -> VOOR.Charging : after(ventpulseWidth,msec)
    VOOR.Charging -> (junction 441) [order 1] : [Mode==2]
    (junction 441) -> VOOR.Pacing : after(Adapted_Interval-ventpulseWidth,msec)
  state AAIR
    state ATRSENSE
      note: Checks if mode has changed
      state Default
        %Exists to check mode and restart timers
      note: If heartbeat detected, waits for
          | falling edge and resets
      note: Waits ARP after sensing or pacing
      state Heartbeat
        %Checks for heartbeat
      note: If no heartbeat after Adapted Interval, send pace
          | so Adapted Rate Limit is met
      state MakeitBeat
        %sends to ventPace
        send(atrpaceStart)%Delivers beat
      (default) -> AAIR.ATRSENSE.Default
      (junction 368) -> AAIR.ATRSENSE.Default : after(atrpulseWidth, msec)
      AAIR.ATRSENSE.Default -> (junction 369) [order 2] : [Mode == 7]
      AAIR.ATRSENSE.Heartbeat -> (junction 368) [order 2] : [AtrDetect==true]
      (junction 369) -> AAIR.ATRSENSE.Heartbeat : after(ARP, msec)
      AAIR.ATRSENSE.Heartbeat -> AAIR.ATRSENSE.MakeitBeat [order 1] : after(Adapted_Interval-ARP,msec)
    note: ATRSENSE:
        | Checks for heartbeat (using sensing in the atrium) after the refractory period, and moves to ATRPACE if no heartbeat is detected.
    state ATRPACE
      state Pacing
        entry:
        PACE_CHARGE_CTRL=false;
        PACE_GND_CTRL=true;
        ATR_PACE_CTRL=true;
        ATR_GND_CTRL=false;
        VENT_GND_CTRL=false;
        VENT_PACE_CTRL=false;
      state Charging
        entry:
        %discharge C21 first
        PACE_GND_CTRL=true;
        VENT_PACE_CTRL=false;
        ATR_PACE_CTRL=false;
        ATR_GND_CTRL=true;
        VENT_GND_CTRL=false;
        %charging C22
        PACING_REF_PWM=atrpulseAmp/5*100;%input from GUI
        PACE_CHARGE_CTRL=true;
        %Return to sensing state
        send(atrPaceEnd);
      note: Drains excess voltage from heart and returns back to sensing
      note: Delivers a pace to the atrium for a duration of the pulse width
      (default) -> AAIR.ATRPACE.Pacing
      AAIR.ATRPACE.Pacing -> AAIR.ATRPACE.Charging : after(atrpulseWidth,msec)
    note: ATRPACE:
        | Sets pins required for atrial pacing (discharging C22), then discharges C21 and recharges C22 before moving back to ATRSENSE.
    (default) -> AAIR.ATRSENSE
    AAIR.ATRSENSE -> AAIR.ATRPACE : atrpaceStart
    AAIR.ATRPACE -> AAIR.ATRSENSE : atrPaceEnd
  note: AAIR:
      | Atrial sensing and pacing
      | at an adapted rate. Detects
      | missed pulses and paces the
      | heart to mantain the required
      | Adapt Rate Interval
  state VVIR
    note: VENTSENSE:
        | Checks for heartbeat (using sensing in the ventricle) after the refractory period, and moves to VENTPACE if no heartbeat is detected.
    state VENTSENSE
      state Default
        LED_STATEB =true;
        %testLED turns on in sensing turns off in pacing
      note: Checks if mode has changed
      note: If natural beat detected, wait until
          | falling edge and reset timing
      note: If correct mode, wait VRP after sense and pace
      state Heartbeat
        %Checks for heartbeat
      note: If no pulse after Adapted Interval is reached, pace heart
      state MakeitBeat
        LED_STATEB = false;
        %sends a beat
        send(ventpaceStart)
      (default) -> VVIR.VENTSENSE.Default
      (junction 316) -> VVIR.VENTSENSE.Default : after(ventpulseWidth, msec)
      VVIR.VENTSENSE.Default -> (junction 317) [order 1] : [Mode == 3]
      VVIR.VENTSENSE.Heartbeat -> (junction 316) [order 1] : [VentDetect == true]
      (junction 317) -> VVIR.VENTSENSE.Heartbeat : after(VRP, msec)
      VVIR.VENTSENSE.Heartbeat -> VVIR.VENTSENSE.MakeitBeat [order 2] : after(Adapted_Interval-VRP, msec)
    state VENTPACE
      state Pacing
        entry:
        PACE_CHARGE_CTRL=false;
        PACE_GND_CTRL=true;
        ATR_PACE_CTRL=false;
        ATR_GND_CTRL=false;
        VENT_GND_CTRL=false;
        VENT_PACE_CTRL=true;
      state Charging
        entry:
        %discharge C21 first
        PACE_GND_CTRL=true;
        VENT_PACE_CTRL=false;
        ATR_PACE_CTRL=false;
        ATR_GND_CTRL=false;
        VENT_GND_CTRL=true;
        %charging C22
        PACING_REF_PWM=ventpulseAmp/5*100;%input from GUI
        PACE_CHARGE_CTRL=true;
        %Return to sensing state
        send(ventPaceEnd);
      note: Drains voltage delivered to allow net charge of 0
      note: Delivers pulse for the duration of pulse width
      (default) -> VVIR.VENTPACE.Pacing
      VVIR.VENTPACE.Pacing -> VVIR.VENTPACE.Charging : after(ventpulseWidth,msec)
    note: VENTPACE:
        | Sets pins required for ventricular pacing (discharging C22), then discharges C21 and recharges C22 before moving back to VENTSENSE.
    (default) -> VVIR.VENTSENSE
    VVIR.VENTSENSE -> VVIR.VENTPACE : ventpaceStart
    VVIR.VENTPACE -> VVIR.VENTSENSE : ventPaceEnd
  note: VVIR:
      | Ventricular sensing and pacing
      | at an adapted rate. Detects
      | missed pulses and paces the
      | heart to mantain the required
      | Adapted Rate Interval
  state AOO
    note: Checks if mode has changed
    state Charging
      entry:
      %discharge C21 first
      PACE_GND_CTRL=true;
      VENT_PACE_CTRL=false;
      Z_ATR_CTRL=false;
      Z_VENT_CTRL=false;
      ATR_PACE_CTRL=false;
      ATR_GND_CTRL=true;
      VENT_GND_CTRL=false;
      %charging C22
      PACING_REF_PWM=atrpulseAmp/5*100;%input from GUI
      PACE_CHARGE_CTRL=true;
      LED_STATEB=true;
    state Pacing
      entry:
      PACE_CHARGE_CTRL=false;
      PACE_GND_CTRL=true;
      ATR_PACE_CTRL=true;
      ATR_GND_CTRL=false;
      Z_ATR_CTRL=false;
      Z_VENT_CTRL=false;
      VENT_GND_CTRL=false;
      VENT_PACE_CTRL=false;
      LED_STATEB=true;
    note: Drains excess current from heart and delivers next pace after LRI
        | in order to meet LRL
    note: Paces atrium for duration of pulse width
    (default) -> AOO.Charging
    AOO.Pacing -> AOO.Charging : after(atrpulseWidth,msec)
    AOO.Charging -> (junction 439) [order 2] : [Mode==4]
    (junction 439) -> AOO.Pacing : after(LRI-atrpulseWidth,msec)
  note: AOO:
      | Atrial pacing at specified rate through discharging C22, discharging C21, and recharging C22.
  note: VOO:
      | Ventricular pacing at specified rate through discharging C22, discharging C21, and recharging C22.
  state VOO
    state Charging
      entry:
      %discharge C21 first at VENT_GND
      PACE_GND_CTRL=true;
      VENT_PACE_CTRL=false;
      Z_ATR_CTRL=false;
      Z_VENT_CTRL=false;
      ATR_PACE_CTRL=false;
      ATR_GND_CTRL=false;
      VENT_GND_CTRL=true;
      %charging C22
      %input from GUI
      PACING_REF_PWM=ventpulseAmp/5*100;
      PACE_CHARGE_CTRL=true;
      LED_STATE=true;
    state Pacing
      entry:
      %discharging C22 at VENT
      PACE_CHARGE_CTRL=false;
      PACE_GND_CTRL=true;
      ATR_PACE_CTRL=false;
      ATR_GND_CTRL=false;
      Z_ATR_CTRL=false;
      Z_VENT_CTRL=false;
      VENT_GND_CTRL=false;
      VENT_PACE_CTRL=true;
      LED_STATE=false;
    note: Checks if mode has changed
    note: Drains excess current from heart and delivers
        |  pace after LRI to meet LRL
    note: Delivers pulse to ventricle for duration of pulse width
    (default) -> VOO.Charging
    VOO.Pacing -> VOO.Charging : after(ventpulseWidth,msec)
    VOO.Charging -> (junction 435) [order 2] : [Mode == 0]
    (junction 435) -> VOO.Pacing : after(LRI-ventpulseWidth,msec)
  state AAI
    state ATRSENSE
      note: Checks if mode has changed
      state Default
        %Exists to check mode and restart timers
      note: If heartbeat detected, waits for
          | falling edge and resets
      note: Waits ARP after sensing or pacing
      state Heartbeat
        %Checks for heartbeat
      note: If no heartbeat after LRI, send pace
          | so LRL is met
      state MakeitBeat
        %sends to ventPace
        send(atrpaceStart)%Delivers beat
      (default) -> AAI.ATRSENSE.Default
      (junction 213) -> AAI.ATRSENSE.Default : after(atrpulseWidth, msec)
      AAI.ATRSENSE.Default -> (junction 359) [order 2] : [Mode == 5]
      AAI.ATRSENSE.Heartbeat -> (junction 213) [order 2] : [AtrDetect==true]
      (junction 359) -> AAI.ATRSENSE.Heartbeat : after(ARP, msec)
      AAI.ATRSENSE.Heartbeat -> AAI.ATRSENSE.MakeitBeat [order 1] : after(LRI-ARP+atrpulseWidth,msec)
    note: ATRSENSE:
        | Checks for heartbeat (using sensing in the atrium) after the refractory period, and moves to ATRPACE if no heartbeat is detected.
    state ATRPACE
      state Pacing
        entry:
        PACE_CHARGE_CTRL=false;
        PACE_GND_CTRL=true;
        ATR_PACE_CTRL=true;
        ATR_GND_CTRL=false;
        VENT_GND_CTRL=false;
        VENT_PACE_CTRL=false;
      state Charging
        entry:
        %discharge C21 first
        PACE_GND_CTRL=true;
        VENT_PACE_CTRL=false;
        ATR_PACE_CTRL=false;
        ATR_GND_CTRL=true;
        VENT_GND_CTRL=false;
        %charging C22
        PACING_REF_PWM=atrpulseAmp/5*100;%input from GUI
        PACE_CHARGE_CTRL=true;
        %Return to sensing state
        send(atrPaceEnd);
      note: Drains excess voltage from heart and returns back to sensing
      note: Delivers a pace to the atrium for a duration of the pulse width
      (default) -> AAI.ATRPACE.Pacing
      AAI.ATRPACE.Pacing -> AAI.ATRPACE.Charging : after(atrpulseWidth,msec)
    note: ATRPACE:
        | Sets pins required for atrial pacing (discharging C22), then discharges C21 and recharges C22 before moving back to ATRSENSE.
    (default) -> AAI.ATRSENSE
    AAI.ATRSENSE -> AAI.ATRPACE : atrpaceStart
    AAI.ATRPACE -> AAI.ATRSENSE : atrPaceEnd
  state VVI
    note: VENTSENSE:
        | Checks for heartbeat (using sensing in the ventricle) after the refractory period, and moves to VENTPACE if no heartbeat is detected.
    state VENTSENSE
      state Default
        LED_STATEB =true;
        %testLED turns on in sensing turns off in pacing
      note: Checks if mode has changed
      note: If natural beat detected, wait until
          | falling edge and reset timing
      note: If correct mode, wait VRP after sense and pace
      state Heartbeat
        %Checks for heartbeat
      note: If no pulse after LRI is reached, pace heart
      state MakeitBeat
        LED_STATEB = false;
        %sends a beat
        send(ventpaceStart)
      (default) -> VVI.VENTSENSE.Default
      (junction 182) -> VVI.VENTSENSE.Default : after(ventpulseWidth, msec)
      VVI.VENTSENSE.Default -> (junction 225) [order 1] : [Mode == 1]
      VVI.VENTSENSE.Heartbeat -> (junction 182) [order 1] : [VentDetect == true]
      (junction 225) -> VVI.VENTSENSE.Heartbeat : after(VRP, msec)
      VVI.VENTSENSE.Heartbeat -> VVI.VENTSENSE.MakeitBeat [order 2] : after(LRI-VRP, msec)
    state VENTPACE
      state Pacing
        entry:
        PACE_CHARGE_CTRL=false;
        PACE_GND_CTRL=true;
        ATR_PACE_CTRL=false;
        ATR_GND_CTRL=false;
        VENT_GND_CTRL=false;
        VENT_PACE_CTRL=true;
      state Charging
        entry:
        %discharge C21 first
        PACE_GND_CTRL=true;
        VENT_PACE_CTRL=false;
        ATR_PACE_CTRL=false;
        ATR_GND_CTRL=false;
        VENT_GND_CTRL=true;
        %charging C22
        PACING_REF_PWM=ventpulseAmp/5*100;%input from GUI
        PACE_CHARGE_CTRL=true;
        %Return to sensing state
        send(ventPaceEnd);
      note: Drains voltage delivered to allow net charge of 0
      note: Delivers pulse for the duration of pulse width
      (default) -> VVI.VENTPACE.Pacing
      VVI.VENTPACE.Pacing -> VVI.VENTPACE.Charging : after(ventpulseWidth,msec)
    note: VENTPACE:
        | Sets pins required for ventricular pacing (discharging C22), then discharges C21 and recharges C22 before moving back to VENTSENSE.
    (default) -> VVI.VENTSENSE
    VVI.VENTSENSE -> VVI.VENTPACE : ventpaceStart
    VVI.VENTPACE -> VVI.VENTSENSE : ventPaceEnd
  note: AAI:
      | Atrial sensing and pacing
      | at a specified rate. Detects
      | missed pulses and paces the
      | heart to mantain the required
      | LRL
  note: VVI:
      | Ventricular sensing and pacing
      | at a specified rate. Detects
      | missed pulses and paces the
      | heart to mantain the required
      | LRL
  AAIR.ATRSENSE.Default -> INITIALIZER [order 1] : [Mode ~= 7]
  AOOR.Charging -> INITIALIZER [order 1] : [Mode ~= 6]
  DOOR.ATR_CHARGING -> INITIALIZER [order 1] : [Mode ~= 9]
  VVI.VENTSENSE.Default -> INITIALIZER [order 2] : [Mode ~= 1]
  AAI.ATRSENSE.Default -> INITIALIZER [order 1] : [Mode ~= 5]
  VOO.Charging -> INITIALIZER [order 1] : [Mode ~= 0]
  DOO.ATR_CHARGING -> INITIALIZER [order 1] : [Mode ~= 8]
  AOO.Charging -> INITIALIZER [order 1] : [Mode ~= 4]
  VVIR.VENTSENSE.Default -> INITIALIZER [order 2] : [Mode ~= 3]
  VOOR.Charging -> INITIALIZER [order 2] : [Mode ~= 2]
  (default) -> INITIALIZER
  INITIALIZER -> DOO [order 1] : [Mode==8]
  INITIALIZER -> DOOR [order 2] : [Mode==9]
  INITIALIZER -> VOOR [order 6] : [Mode==2]
  INITIALIZER -> AOOR [order 5] : [Mode==6]
  INITIALIZER -> AAIR [order 3] : [Mode == 7]
  INITIALIZER -> VVIR [order 8] : [Mode==3]
  INITIALIZER -> AOO [order 9] : [Mode==4]
  INITIALIZER -> VOO [order 7] : [Mode==0]
  INITIALIZER -> AAI [order 4] : [Mode == 5]
  INITIALIZER -> VVI [order 10] : [Mode==1]
  data: PVARP input; AtrDetect input boolean; ventpulseAmp input; AV_Delay input; VentDetect input boolean; Mode input; VRP input; ARP input; atrpulseWidth input; ventpulseWidth input; Adapted_Interval input double; LRI input double; atrpulseAmp input; Z_ATR_CTRL output; Z_VENT_CTRL output; PACING_REF_PWM output; ATR_PACE_CTRL output; VENT_PACE_CTRL output; PACE_GND_CTRL output; ATR_GND_CTRL output; VENT_GND_CTRL output; PACE_CHARGE_CTRL output; LED_STATE output; LED_STATEB output; Natural_Beat local; Nat_Vent local; Nat_Atr local; Rate local
  events: paceEnd local FUNCTION_CALL_EVENT; paceStart local FUNCTION_CALL_EVENT; ventpaceStart local FUNCTION_CALL_EVENT; atrpaceStart local FUNCTION_CALL_EVENT; ventPaceEnd local FUNCTION_CALL_EVENT; atrPaceEnd local FUNCTION_CALL_EVENT

== stateflow chart Pacemaker/Inputs/COM_IN ==
  settings: executeAtInitialization=1
  state Set_Params
    entry:
    MODE = typecast(RX_D(3:4), 'uint16');
    LRL = typecast(RX_D(5:6), 'uint16');
    URL = typecast(RX_D(7:8), 'uint16');
    MAX_SENSE = typecast(RX_D(9:10), 'uint16');
    AV_DELAY = typecast(RX_D(11:12), 'uint16');
    ATR_AMP = typecast(RX_D(13:20), 'double');
    ATR_PW = typecast(RX_D(21:22), 'uint16');
    ATR_SENSE = typecast(RX_D(23:30), 'double');
    VENT_AMP = typecast(RX_D(31:38), 'double');
    VENT_PW = typecast(RX_D(39:40), 'uint16');
    VENT_SENSE = typecast(RX_D(41:48), 'double');
    ARP = typecast(RX_D(49:50), 'uint16');
    VRP = typecast(RX_D(51:52), 'uint16');
    PVARP = typecast(RX_D(53:54), 'uint16');
    ACTIVITY_THRESH = typecast(RX_D(55:62), 'double');
    REACT_TIME = typecast(RX_D(63:64), 'uint16');
    RESP_FACTOR = typecast(RX_D(65:66), 'uint16');
    RCVR_TIME = typecast(RX_D(67:68), 'uint16');
    Send_Params_To_DCMMM();
  state Initial
    % Set initial values of parameter
    entry:
    MODE = 1;
    LRL = 60;
    URL = 120;
    PVARP = 200;
    AV_DELAY = 40;
    REACT_TIME = 30;
    RESP_FACTOR = 16;
    ACTIVITY_THRESH = 1;
    RCVR_TIME = 5;
    MAX_SENSE = 120;
    ATR_AMP = 4;
    ATR_PW = 20;
    ARP = 200;
    ATR_SENSE = 3;
    VENT_AMP = 4;
    VENT_PW = 10;
    VRP = 200;
    VENT_SENSE = 3;
  state Standby
    % Waiting for COM
  state Echo_Params
    entry:
    Send_Params_To_DCMMM();
  Set_Params -> Standby
  (default) -> Initial
  (junction 15) -> Set_Params [order 1] : [RX_D(2) == hex2dec('55')]
  (junction 13) -> Standby [order 2]
  Initial -> Standby
  Standby -> (junction 13) : [Status == 0]
  (junction 13) -> (junction 15) [order 1] : [RX_D(1) == hex2dec('16')]
  (junction 15) -> Echo_Params [order 2] : [RX_D(2) == hex2dec('22')]
  Echo_Params -> Standby
  data: RX_D input uint8; Status input uint8; MODE output uint16; LRL output uint16; URL output uint16; MAX_SENSE output uint16; AV_DELAY output uint16; ATR_AMP output double; ATR_PW output uint16; ATR_SENSE output double; VENT_AMP output double; VENT_PW output uint16; VENT_SENSE output double; ARP output uint16; VRP output uint16; PVARP output uint16; ACTIVITY_THRESH output double; REACT_TIME output uint16; RESP_FACTOR output uint16; RCVR_TIME output uint16
